simulink model "Steinwurf"  (Simulink 7.1)
settings: Solver=ode45  StartTime=0.0  StopTime=1.4  RelTol=1e-3
settings Model: Creator=Meisel  LastModifiedBy=Meisel

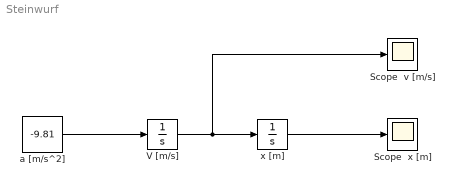
== system Steinwurf ==
  Scope  v [m/s] : Scope
  Scope  x [m] : Scope
  V [m/s] : Integrator  InitialCondition=5
  a [m/s^2] : Constant  Value=-9.81  OutDataType=sfix(16)  OutScaling=2^0
  x [m] : Integrator  InitialCondition=1.2
  wires:
  a [m/s^2]/1 -> V [m/s]/1
  V [m/s]/1 -> x [m]/1, Scope  v [m/s]/1
  x [m]/1 -> Scope  x [m]/1
